simulink model "SAME70Q21B_MCLV2_LongHurstMotor_WithEncoder"  (R2018a)
settings: Solver=FixedStepDiscrete  StartTime=0.0  StopTime=10.0  FixedStep=50e-6  RelTol=1e-3  EnableMultiTasking=on
undefined symbols (not defined in the file or in its folder): A24, DiscIntNeverNeededParam, LQFP144, MaxPer, ms, ns, PA0, PA1, PA10, PA11, PA12, PA13, PA9, PD18, PD19, PD24, PD25, PD26, Pin, PWM1max, Resol, SAME70Q21B, Timer
libraries: MCHP_Blockset x10, simulink x5
(part 2 of 2)

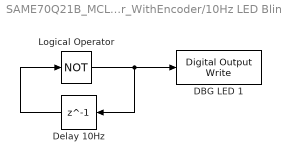
== system SAME70Q21B_MCLV2_LongHurstMotor_WithEncoder/10Hz LED Blink ==
  DBG LED 1 : MCHP_Blockset/Digital IO/Digital Output Write  PORT=Dynamic Options  PORT_TXT="C   [ 0 : 31 ]"  PIN=23  PACK=off  SIMULTANEOUS=off  ORDERING=None  SampleTime=-1  MCHP_PORT={Digital Out}{DOU}1:1:C23;  MCHP_MASTERLINK=SAME70Q21B_MCLV2_LongHurstMotor_WithEncoder/Microchip Master
      settings: SourceProductName=MPLAB Device Blocks for Simulink
  Delay 10Hz : Delay  DelayLength=1  InitialCondition=0  SampleTime=.05
  Logical Operator : Logic  Operator=NOT  AllPortsSameDT=off  OutDataTypeStr=boolean
  wires:
  Logical Operator/1 -> DBG LED 1/1, Delay 10Hz/1
  Delay 10Hz/1 -> Logical Operator/1

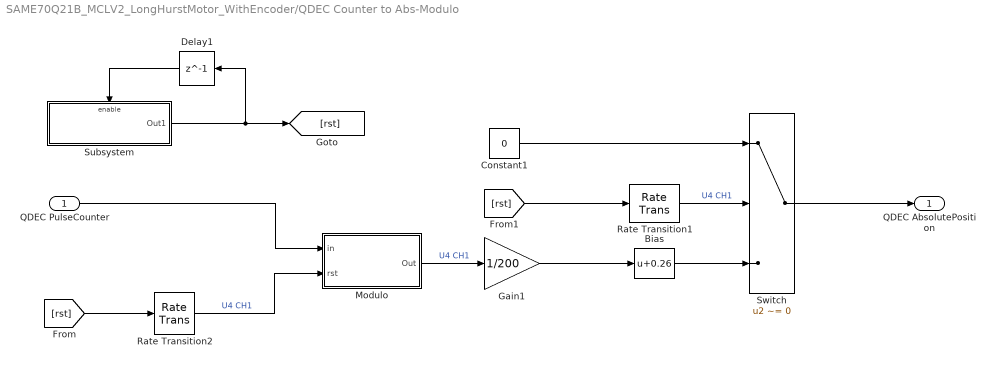
== system SAME70Q21B_MCLV2_LongHurstMotor_WithEncoder/QDEC Counter to Abs-Modulo ==
  QDEC PulseCounter : Inport
  Bias : Bias  Bias=0.26
  Constant1 : Constant  Value=0  OutDataTypeStr=Inherit: Inherit via back propagation  SampleTime=-1
  Delay1 : Delay  DelayLength=1  InitialCondition=1
  Gain1 : Gain  Gain=1/200  OutDataTypeStr=fixdt(0,32,32)
  Modulo : Subsystem
  Rate Transition1 : RateTransition  Deterministic=off
  Rate Transition2 : RateTransition  Deterministic=off
  Subsystem : Subsystem
  Switch : Switch  Criteria=u2 ~= 0
  QDEC AbsolutePosition : Outport  VectorParamsAs1DForOutWhenUnconnected=off
  wires:
  Gain1/1 -> Bias/1
  Delay1/1 -> Subsystem/Enable
  [rst] -> Rate Transition2/1
  Modulo/1(Out) -> Gain1/1  "U4 CH1"
  Subsystem/1(Out1) -> Delay1/1, [rst]
  [rst] -> Rate Transition1/1
  Bias/1 -> Switch/3
  Rate Transition1/1 -> Switch/2  "U4 CH1"
  Rate Transition2/1 -> Modulo/2(rst)  "U4 CH1"
  Constant1/1 -> Switch/1
  QDEC PulseCounter/1 -> Modulo/1(in)
  Switch/1 -> QDEC AbsolutePosition/1

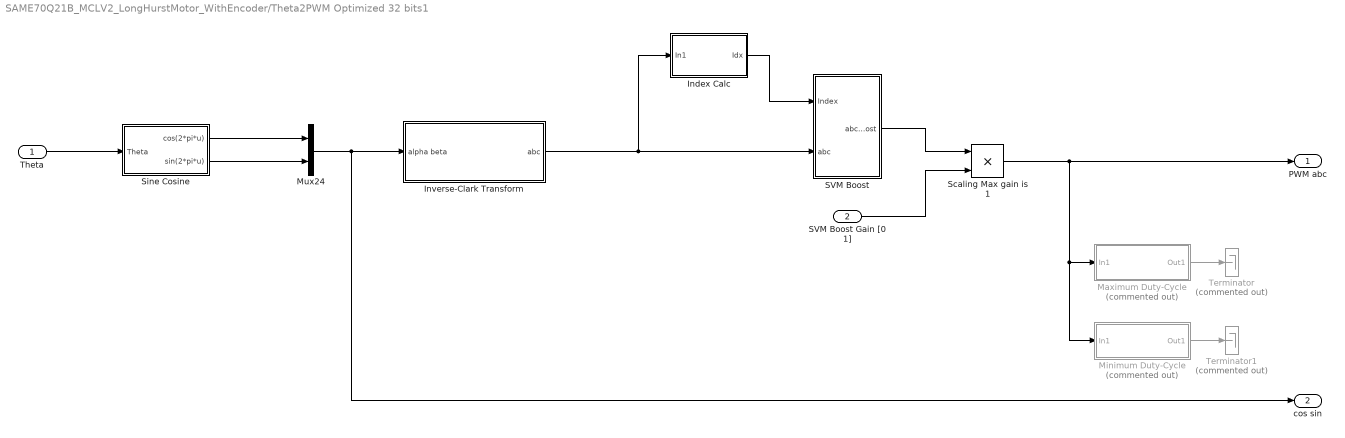
== system SAME70Q21B_MCLV2_LongHurstMotor_WithEncoder/Theta2PWM Optimized 32 bits1 ==
  Theta : Inport
  SVM Boost Gain [0 1] : Inport  Port=2  OutMax=1
  Index Calc : Subsystem
  Inverse-Clark Transform : Subsystem
  Maximum Duty-Cycle : Subsystem  Commented=on
  Minimum Duty-Cycle : Subsystem  Commented=on
  Mux24 : Mux  Inputs=2
  SVM Boost : Subsystem
  Scaling Max gain is 1 : Product  Inputs=**  OutDataTypeStr=single
  Sine Cosine : Subsystem
  Terminator : Terminator  Commented=on
  Terminator1 : Terminator  Commented=on
  PWM abc : Outport  VectorParamsAs1DForOutWhenUnconnected=off
  cos sin : Outport  Port=2  VectorParamsAs1DForOutWhenUnconnected=off
  wires:
  Mux24/1 -> cos sin/1, Inverse-Clark Transform/1(alpha beta)
  SVM Boost/1(abc boost) -> Scaling Max gain is 1/1
  Sine Cosine/2(sin(2*pi*u)) -> Mux24/2
  Sine Cosine/1(cos(2*pi*u)) -> Mux24/1
  Theta/1 -> Sine Cosine/1(Theta)
  Inverse-Clark Transform/1(abc) -> SVM Boost/2(abc), Index Calc/1(In1)
  Index Calc/1(Idx) -> SVM Boost/1(Index)
  SVM Boost Gain [0 1]/1 -> Scaling Max gain is 1/2
  Maximum Duty-Cycle/1(Out1) -> Terminator/1
  Minimum Duty-Cycle/1(Out1) -> Terminator1/1
  Scaling Max gain is 1/1 -> PWM abc/1, Maximum Duty-Cycle/1(In1), Minimum Duty-Cycle/1(In1)

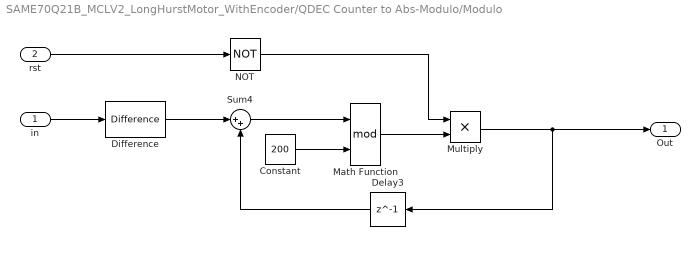
== system SAME70Q21B_MCLV2_LongHurstMotor_WithEncoder/QDEC Counter to Abs-Modulo/Modulo ==
  in : Inport
  rst : Inport  Port=2  OutDataTypeStr=boolean
  Constant : Constant  Value=200  OutDataTypeStr=Inherit: Inherit via back propagation
  Delay3 : Delay  DelayLength=1  InitialCondition=0
  Difference : simulink/Discrete/Difference  ICPrevInput=0  OutMin=[]  OutMax=[]  OutDataTypeStr=int16  OutputDataTypeScalingMode=int16  OutDataType=fixdt(1, 16)  OutScaling=2^-10  DoSatur=off
  Math Function : Math  Operator=mod  SaturateOnIntegerOverflow=on
  Multiply : Product  OutDataTypeStr=uint16
  NOT : Logic  Operator=NOT  IconShape=distinctive  AllPortsSameDT=off  OutDataTypeStr=boolean
  Sum4 : Sum  Inputs=|++  OutDataTypeStr=Inherit: Same as first input
  Out : Outport  VectorParamsAs1DForOutWhenUnconnected=off
  wires:
  Sum4/1 -> Math Function/1
  Constant/1 -> Math Function/2
  Delay3/1 -> Sum4/2
  Difference/1 -> Sum4/1
  rst/1 -> NOT/1
  Math Function/1 -> Multiply/2
  Multiply/1 -> Delay3/1, Out/1
  NOT/1 -> Multiply/1
  in/1 -> Difference/1

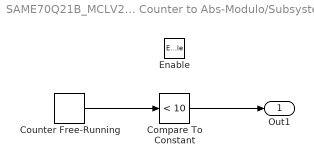
== system SAME70Q21B_MCLV2_LongHurstMotor_WithEncoder/QDEC Counter to Abs-Modulo/Subsystem ==
  Enable : EnablePort
  Compare To Constant : simulink/Logic and Bit Operations/Compare To Constant  relop=<  const=10  OutDataTypeStr=boolean
  Counter Free-Running : simulink/Sources/Counter Free-Running  NumBits=16  tsamp=.1
  Out1 : Outport  VectorParamsAs1DForOutWhenUnconnected=off
  wires:
  Counter Free-Running/1 -> Compare To Constant/1
  Compare To Constant/1 -> Out1/1

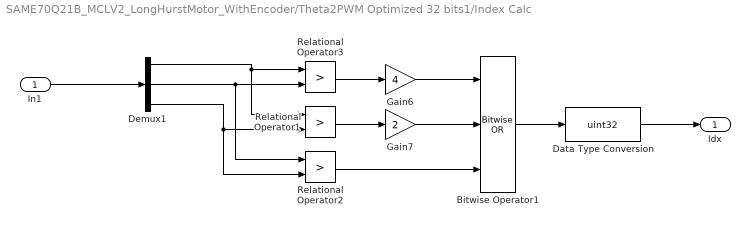
== system SAME70Q21B_MCLV2_LongHurstMotor_WithEncoder/Theta2PWM Optimized 32 bits1/Index Calc ==
  In1 : Inport
  Bitwise Operator1 : simulink/Logic and Bit Operations/Bitwise Operator  logicop=OR  UseBitMask=off  NumInputPorts=3  BitMask=bin2dec('11011001')  BitMaskRealWorld=Stored Integer
  Data Type Conversion : DataTypeConversion  OutDataTypeStr=uint32  ConvertRealWorld=Stored Integer (SI)
  Demux1 : Demux  Outputs=3
  Gain6 : Gain  Gain=4  OutDataTypeStr=Inherit: Same as input
  Gain7 : Gain  Gain=2  OutDataTypeStr=Inherit: Same as input
  Relational Operator1 : RelationalOperator  Operator=>  OutDataTypeStr=fixdt(0,32)  RndMeth=Nearest
  Relational Operator2 : RelationalOperator  Operator=>  OutDataTypeStr=fixdt(0,32)  RndMeth=Nearest
  Relational Operator3 : RelationalOperator  Operator=>  OutDataTypeStr=fixdt(0,32)  RndMeth=Nearest
  Idx : Outport  VectorParamsAs1DForOutWhenUnconnected=off
  wires:
  Data Type Conversion/1 -> Idx/1
  In1/1 -> Demux1/1
  Bitwise Operator1/1 -> Data Type Conversion/1
  Demux1/1 -> Relational Operator1/1, Relational Operator3/1
  Relational Operator1/1 -> Gain7/1
  Demux1/3 -> Relational Operator1/2, Relational Operator2/2
  Demux1/2 -> Relational Operator3/2, Relational Operator2/1
  Relational Operator3/1 -> Gain6/1
  Relational Operator2/1 -> Bitwise Operator1/3
  Gain6/1 -> Bitwise Operator1/1
  Gain7/1 -> Bitwise Operator1/2

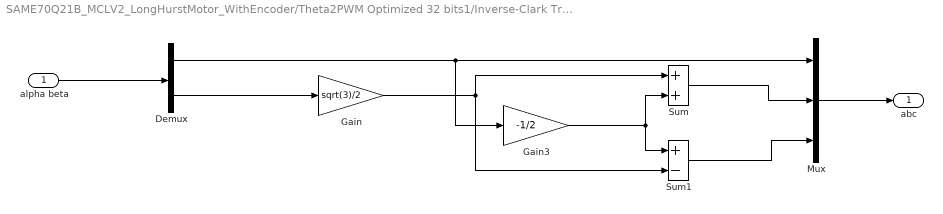
== system SAME70Q21B_MCLV2_LongHurstMotor_WithEncoder/Theta2PWM Optimized 32 bits1/Inverse-Clark Transform ==
  alpha beta : Inport
  Demux : Demux  Outputs=2
  Gain : Gain  Gain=sqrt(3)/2  OutDataTypeStr=Inherit: Inherit via back propagation  RndMeth=Zero
  Gain3 : Gain  Gain=-1/2  OutDataTypeStr=Inherit: Inherit via back propagation  RndMeth=Zero
  Mux : Mux  Inputs=3
  Sum : Sum  RndMeth=Zero  OutDataTypeStr=Inherit: Same as first input
  Sum1 : Sum  Inputs=+-  RndMeth=Zero  SaturateOnIntegerOverflow=on  OutDataTypeStr=Inherit: Same as first input
  abc : Outport  VectorParamsAs1DForOutWhenUnconnected=off
  wires:
  Demux/1 -> Gain3/1, Mux/1
  Demux/2 -> Gain/1
  alpha beta/1 -> Demux/1
  Gain/1 -> Sum1/2, Sum/1
  Sum/1 -> Mux/2
  Sum1/1 -> Mux/3
  Gain3/1 -> Sum/2, Sum1/1
  Mux/1 -> abc/1

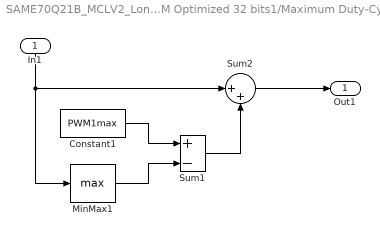
== system SAME70Q21B_MCLV2_LongHurstMotor_WithEncoder/Theta2PWM Optimized 32 bits1/Maximum Duty-Cycle ==
  In1 : Inport
  Constant1 : Constant  Value=PWM1max  OutDataTypeStr=uint16
  MinMax1 : MinMax  Function=max  InputSameDT=on  OutDataTypeStr=int16
  Sum1 : Sum  Inputs=+-  AccumDataTypeStr=uint16  OutDataTypeStr=Inherit: Same as accumulator  RndMeth=Simplest
  Sum2 : Sum  Inputs=|++  AccumDataTypeStr=uint16  OutDataTypeStr=Inherit: Same as accumulator  RndMeth=Simplest
  Out1 : Outport  VectorParamsAs1DForOutWhenUnconnected=off
  wires:
  Constant1/1 -> Sum1/1
  MinMax1/1 -> Sum1/2
  In1/1 -> Sum2/1, MinMax1/1
  Sum2/1 -> Out1/1
  Sum1/1 -> Sum2/2

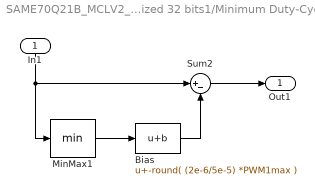
== system SAME70Q21B_MCLV2_LongHurstMotor_WithEncoder/Theta2PWM Optimized 32 bits1/Minimum Duty-Cycle ==
  In1 : Inport
  Bias : Bias  Bias=-round( (2e-6/5e-5) *PWM1max )
  MinMax1 : MinMax  InputSameDT=on  OutDataTypeStr=int16
  Sum2 : Sum  Inputs=|+-  AccumDataTypeStr=uint16  OutDataTypeStr=Inherit: Same as accumulator  RndMeth=Simplest
  Out1 : Outport  VectorParamsAs1DForOutWhenUnconnected=off
  wires:
  In1/1 -> MinMax1/1, Sum2/1
  Sum2/1 -> Out1/1
  MinMax1/1 -> Bias/1
  Bias/1 -> Sum2/2

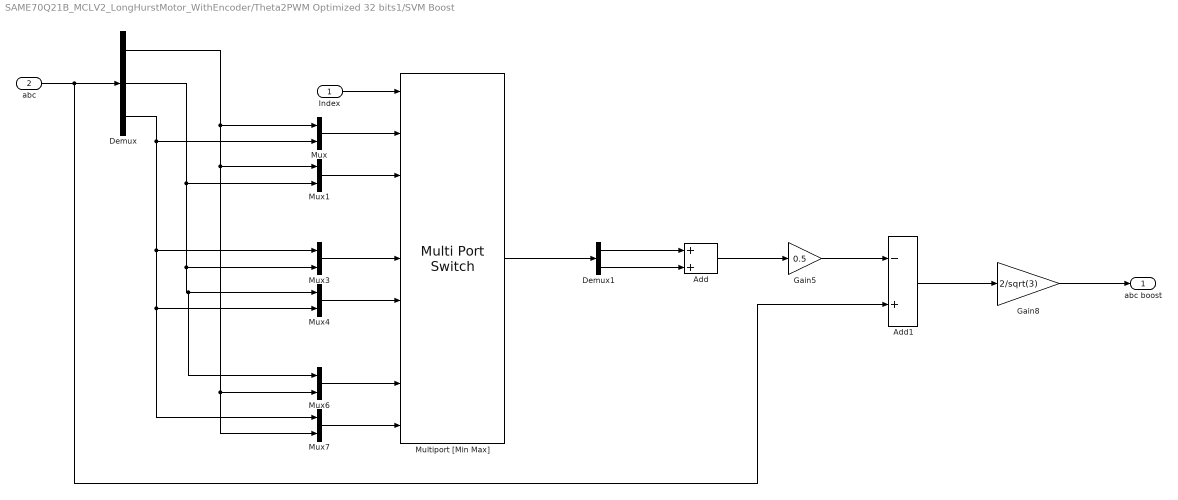
== system SAME70Q21B_MCLV2_LongHurstMotor_WithEncoder/Theta2PWM Optimized 32 bits1/SVM Boost ==
  Index : Inport
  abc : Inport  Port=2
  Add : Sum  OutDataTypeStr=Inherit: Same as accumulator  RndMeth=Zero
  Add1 : Sum  Inputs=-+  RndMeth=Zero  OutDataTypeStr=Inherit: Same as first input
  Demux : Demux  Outputs=3
  Demux1 : Demux  Outputs=2
  Gain5 : Gain  Gain=0.5  RndMeth=Zero  OutDataTypeStr=Inherit: Same as input
  Gain8 : Gain  Gain=2/sqrt(3)  RndMeth=Zero  ParamDataTypeStr=Inherit: Same as input
  Multiport [Min Max] : MultiPortSwitch  DataPortOrder=Zero-based contiguous  Inputs=8  DiagnosticForDefault=None  zeroidx=on
  Mux{,1,3..4,6..7} (6 alike) : Mux  Inputs=2
  abc boost : Outport  VectorParamsAs1DForOutWhenUnconnected=off
  wires:
  Add/1 -> Gain5/1
  Gain5/1 -> Add1/1
  Add1/1 -> Gain8/1
  abc/1 -> Add1/2, Demux/1
  Gain8/1 -> abc boost/1
  Index/1 -> Multiport [Min Max]/1
  Mux/1 -> Multiport [Min Max]/2
  Mux1/1 -> Multiport [Min Max]/3
  Mux3/1 -> Multiport [Min Max]/5
  Mux4/1 -> Multiport [Min Max]/6
  Mux6/1 -> Multiport [Min Max]/8
  Mux7/1 -> Multiport [Min Max]/9
  Demux/1 -> Mux7/2, Mux6/2, Mux1/1, Mux/1
  Demux/3 -> Mux/2, Mux3/1, Mux4/2, Mux7/1
  Demux/2 -> Mux6/1, Mux4/1, Mux3/2, Mux1/2
  Multiport [Min Max]/1 -> Demux1/1
  Demux1/1 -> Add/1
  Demux1/2 -> Add/2

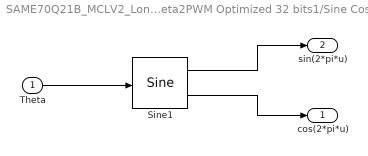
== system SAME70Q21B_MCLV2_LongHurstMotor_WithEncoder/Theta2PWM Optimized 32 bits1/Sine Cosine ==
  Theta : Inport
  Sine1 : simulink/Lookup Tables/Sine  Formula=sin(2*pi*u) and cos(2*pi*u)  NumDataPoints=(2^5)+1  OutputWordLength=16  InternalRulePriority=Speed
  cos(2*pi*u) : Outport  VectorParamsAs1DForOutWhenUnconnected=off
  sin(2*pi*u) : Outport  Port=2  VectorParamsAs1DForOutWhenUnconnected=off
  wires:
  Theta/1 -> Sine1/1
  Sine1/1 -> sin(2*pi*u)/1
  Sine1/2 -> cos(2*pi*u)/1
